simulink model "Simulator_Case_1"  (R2024a)
settings: Solver=VariableStepAuto  StartTime=0.0  StopTime=2842  RelTol=1e-3
values from neighbouring files (symbols this model uses):
  Position_Initial_X = Waypoints_X(1)    [Parametrization_Simulation_Case_1.m]
  Position_Initial_Y = Waypoints_Y(1)    [Parametrization_Simulation_Case_1.m]
undefined symbols (not defined in the file or in its folder): Gain_Derivative_Controller, Gain_Integral_Controller, Gain_Proportional_Controller, Velocity_Ship_Mean, Waypoints
libraries: cstblocks x2
settings Model: Creator=gerar  LastModifiedBy=gerar

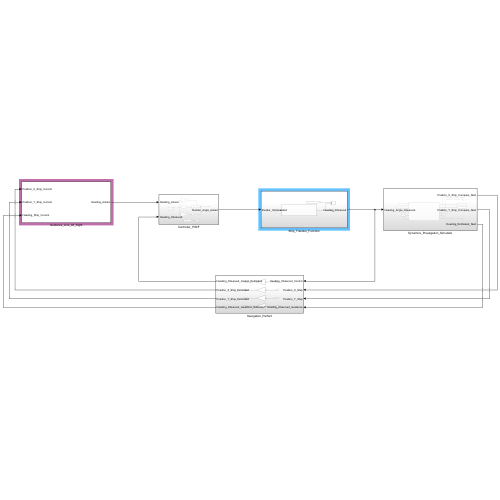
[thumbnail: Simulink's stored preview of the top-level diagram]
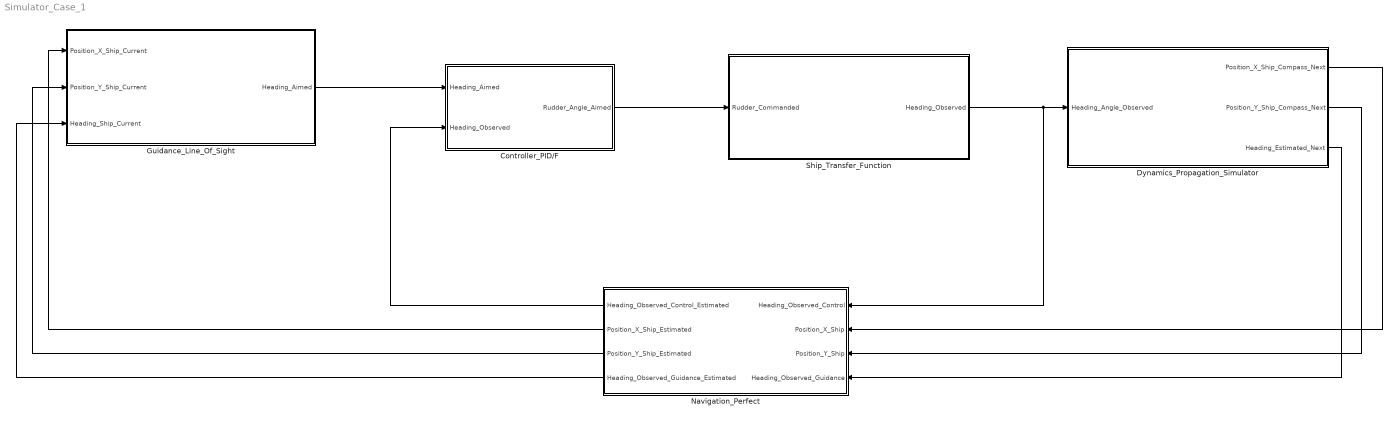
== system Simulator_Case_1 ==
  Controller_PID/F : Subsystem
  Dynamics_Propagation_Simulator : Subsystem
  Guidance_Line_Of_Sight : Subsystem
  Navigation_Perfect : Subsystem
  Ship_Transfer_Function : Subsystem
  wires:
  Guidance_Line_Of_Sight/1(Heading_Aimed) -> Controller_PID/F/1(Heading_Aimed)
  Controller_PID/F/1(Rudder_Angle_Aimed) -> Ship_Transfer_Function/1(Rudder_Commanded)
  Ship_Transfer_Function/1(Heading_Observed) -> Navigation_Perfect/1(Heading_Observed_Control), Dynamics_Propagation_Simulator/1(Heading_Angle_Observed)
  Navigation_Perfect/1(Heading_Observed_Control_Estimated) -> Controller_PID/F/2(Heading_Observed)
  Navigation_Perfect/2(Position_X_Ship_Estimated) -> Guidance_Line_Of_Sight/1(Position_X_Ship_Current)
  Navigation_Perfect/3(Position_Y_Ship_Estimated) -> Guidance_Line_Of_Sight/2(Position_Y_Ship_Current)
  Navigation_Perfect/4(Heading_Observed_Guidance_Estimated) -> Guidance_Line_Of_Sight/3(Heading_Ship_Current)
  Dynamics_Propagation_Simulator/1(Position_X_Ship_Compass_Next) -> Navigation_Perfect/2(Position_X_Ship)
  Dynamics_Propagation_Simulator/2(Position_Y_Ship_Compass_Next) -> Navigation_Perfect/3(Position_Y_Ship)
  Dynamics_Propagation_Simulator/3(Heading_Estimated_Next) -> Navigation_Perfect/4(Heading_Observed_Guidance)

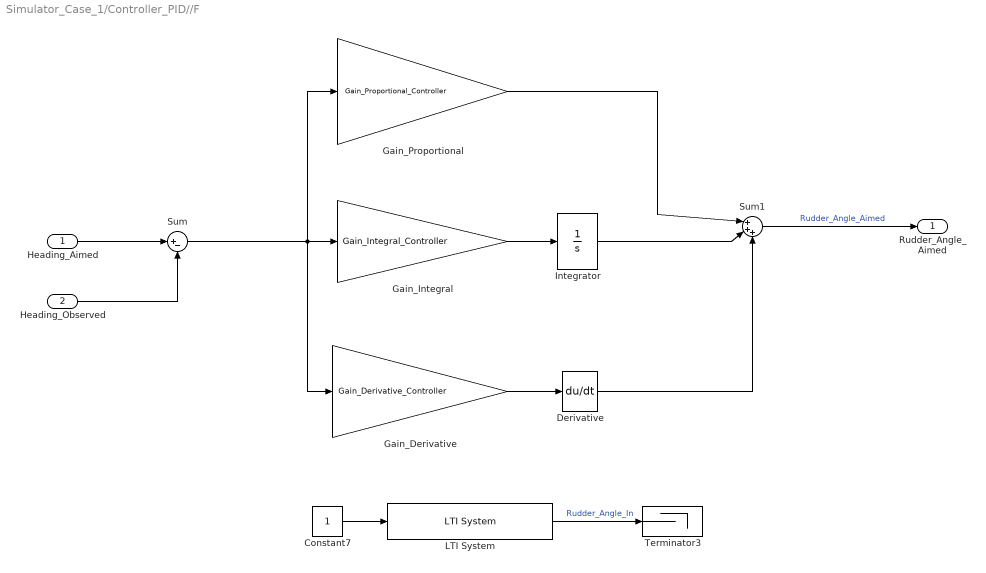
== system Simulator_Case_1/Controller_PID//F ==
  Heading_Aimed : Inport
  Heading_Observed : Inport  Port=2
  Constant7 : Constant
  Derivative : Derivative
  Gain_Derivative : Gain  Gain=Gain_Derivative_Controller
  Gain_Integral : Gain  Gain=Gain_Integral_Controller
  Gain_Proportional : Gain  Gain=Gain_Proportional_Controller
  Integrator : Integrator
  LTI System : cstblocks/LTI System  sys=Controller_PIDF  IC=[]  PadeOrder=0
  Sum : Sum  Inputs=|+-
  Sum1 : Sum  Inputs=|+++
  Terminator3 : Terminator
  Rudder_Angle_Aimed : Outport
  wires:
  Sum/1 -> Gain_Proportional/1, Gain_Integral/1, Gain_Derivative/1
  Gain_Integral/1 -> Integrator/1
  Sum1/1 -> Rudder_Angle_Aimed/1  "Rudder_Angle_Aimed"
  Gain_Proportional/1 -> Sum1/1
  Gain_Derivative/1 -> Derivative/1
  Derivative/1 -> Sum1/3
  Integrator/1 -> Sum1/2
  Heading_Aimed/1 -> Sum/1
  Heading_Observed/1 -> Sum/2
  LTI System/1 -> Terminator3/1  "Rudder_Angle_In"
  Constant7/1 -> LTI System/1

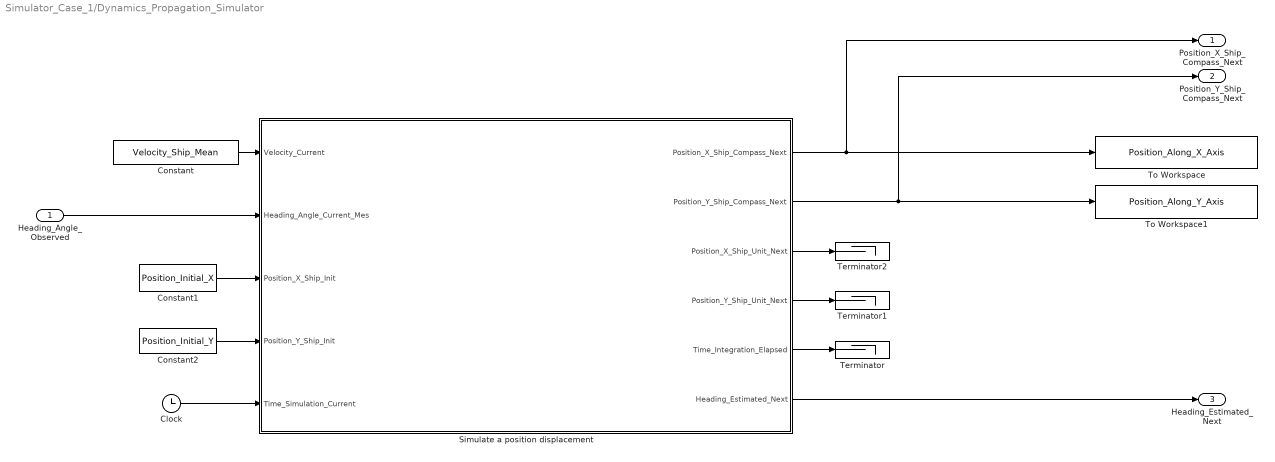
== system Simulator_Case_1/Dynamics_Propagation_Simulator ==
  Heading_Angle_Observed : Inport
  Clock : Clock
  Constant : Constant  Value=Velocity_Ship_Mean
  Constant1 : Constant  Value=Position_Initial_X
  Constant2 : Constant  Value=Position_Initial_Y
  Simulate a position displacement : MATLAB Function  TreatAsAtomicUnit=on
  Terminator : Terminator
  Terminator1 : Terminator
  Terminator2 : Terminator
  To Workspace : ToWorkspace  VariableName=Position_Along_X_Axis  SaveFormat=Timeseries  SampleTime=-1
  To Workspace1 : ToWorkspace  VariableName=Position_Along_Y_Axis  SaveFormat=Timeseries  SampleTime=-1
  Position_X_Ship_Compass_Next : Outport
  Position_Y_Ship_Compass_Next : Outport  Port=2
  Heading_Estimated_Next : Outport  Port=3
  wires:
  Simulate a position displacement/1(Position_X_Ship_Compass_Next) -> Position_X_Ship_Compass_Next/1, To Workspace/1
  Heading_Angle_Observed/1 -> Simulate a position displacement/2(Heading_Angle_Current_Mes)
  Simulate a position displacement/5(Time_Integration_Elapsed) -> Terminator/1
  Simulate a position displacement/4(Position_Y_Ship_Unit_Next) -> Terminator1/1
  Constant1/1 -> Simulate a position displacement/3(Position_X_Ship_Init)
  Constant/1 -> Simulate a position displacement/1(Velocity_Current)
  Simulate a position displacement/2(Position_Y_Ship_Compass_Next) -> Position_Y_Ship_Compass_Next/1, To Workspace1/1
  Simulate a position displacement/3(Position_X_Ship_Unit_Next) -> Terminator2/1
  Constant2/1 -> Simulate a position displacement/4(Position_Y_Ship_Init)
  Clock/1 -> Simulate a position displacement/5(Time_Simulation_Current)
  Simulate a position displacement/6(Heading_Estimated_Next) -> Heading_Estimated_Next/1

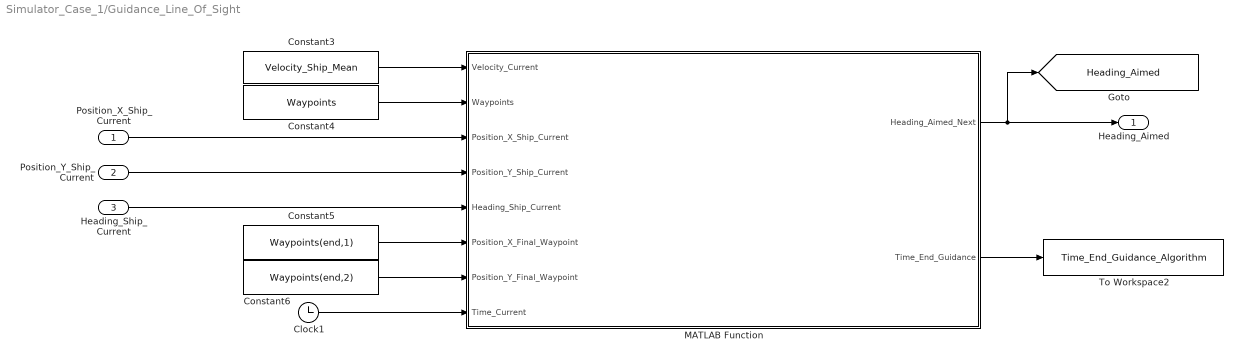
== system Simulator_Case_1/Guidance_Line_Of_Sight ==
  Position_X_Ship_Current : Inport
  Position_Y_Ship_Current : Inport  Port=2
  Heading_Ship_Current : Inport  Port=3
  Clock1 : Clock
  Constant3 : Constant  Value=Velocity_Ship_Mean
  Constant4 : Constant  Value=Waypoints
  Constant5 : Constant  Value=Waypoints(end,1)
  Constant6 : Constant  Value=Waypoints(end,2)
  MATLAB Function : MATLAB Function  TreatAsAtomicUnit=on
  To Workspace2 : ToWorkspace  VariableName=Time_End_Guidance_Algorithm  SaveFormat=Timeseries  SampleTime=-1
  Heading_Aimed : Outport
  tag scope: Heading_Aimed=global
  wires:
  Constant5/1 -> MATLAB Function/6(Position_X_Final_Waypoint)
  Position_X_Ship_Current/1 -> MATLAB Function/3(Position_X_Ship_Current)
  MATLAB Function/1(Heading_Aimed_Next) -> [Heading_Aimed], Heading_Aimed/1
  Constant4/1 -> MATLAB Function/2(Waypoints)
  Constant3/1 -> MATLAB Function/1(Velocity_Current)
  Constant6/1 -> MATLAB Function/7(Position_Y_Final_Waypoint)
  Clock1/1 -> MATLAB Function/8(Time_Current)
  Position_Y_Ship_Current/1 -> MATLAB Function/4(Position_Y_Ship_Current)
  Heading_Ship_Current/1 -> MATLAB Function/5(Heading_Ship_Current)
  MATLAB Function/2(Time_End_Guidance) -> To Workspace2/1

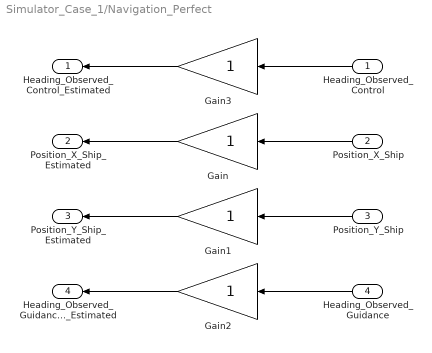
== system Simulator_Case_1/Navigation_Perfect ==
  Heading_Observed_Control : Inport
  Position_X_Ship : Inport  Port=2
  Position_Y_Ship : Inport  Port=3
  Heading_Observed_Guidance : Inport  Port=4
  Gain{,1..3} (4 alike) : Gain
  Heading_Observed_Control_Estimated : Outport
  Position_X_Ship_Estimated : Outport  Port=2
  Position_Y_Ship_Estimated : Outport  Port=3
  Heading_Observed_Guidance_Estimated : Outport  Port=4
  wires:
  Gain1/1 -> Position_Y_Ship_Estimated/1
  Position_X_Ship/1 -> Gain/1
  Heading_Observed_Guidance/1 -> Gain2/1
  Heading_Observed_Control/1 -> Gain3/1
  Gain2/1 -> Heading_Observed_Guidance_Estimated/1
  Position_Y_Ship/1 -> Gain1/1
  Gain/1 -> Position_X_Ship_Estimated/1
  Gain3/1 -> Heading_Observed_Control_Estimated/1

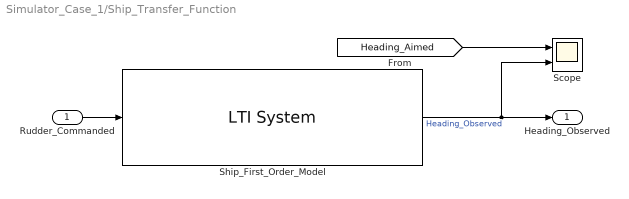
== system Simulator_Case_1/Ship_Transfer_Function ==
  Rudder_Commanded : Inport
  Scope : Scope  NumInputPorts=2
  Ship_First_Order_Model : cstblocks/LTI System  sys=Heading_On_Rudder_Transfer_First_Order  IC=[]  PadeOrder=0
  Heading_Observed : Outport
  wires:
  Ship_First_Order_Model/1 -> Scope/2, Heading_Observed/1  "Heading_Observed"
  Rudder_Commanded/1 -> Ship_First_Order_Model/1
  [Heading_Aimed] -> Scope/1

== matlab function Simulator_Case_1/Guidance_Line_Of_Sight/MATLAB Function ==
  settings: updateMethod=DISCRETE
  data: Velocity_Current input; Heading_Aimed_Next output; Waypoints input; Position_X_Ship_Current input; Position_Y_Ship_Current input; Heading_Ship_Current input; Position_X_Final_Waypoint input; Position_Y_Final_Waypoint input; Time_Current input; Time_End_Guidance output
function [Heading_Aimed_Next,Time_End_Guidance] = Guidance_Waypoints_Following(Velocity_Current,...
                                                                               Waypoints,...
                                                                               Position_X_Ship_Current,...
                                                                               Position_Y_Ship_Current,...
                                                                               Heading_Ship_Current,...
                                                                               Position_X_Final_Waypoint,...
                                                                               Position_Y_Final_Waypoint,...
                                                                               Time_Current)

% Terminal point features:
Position_X_Final_Point = Position_X_Final_Waypoint;
Position_Y_Final_Point = Position_Y_Final_Waypoint;
Radius_Final_Waypoint = 50;

% Enable Guidance to work if the ship is not close to the final waypoint:
if ~((Position_X_Ship_Current - Position_X_Final_Point)^2 + (Position_Y_Ship_Current - Position_Y_Final_Point)^2 <= Radius_Final_Waypoint^2)

    % Then settle the time of end Guidance:
    Time_End_Guidance = 0;

    % Retreive the aimed heading angle that must be performed at this step time
    % of the simulation to follow the Waypoints generated trajectory:
    [Heading_Aimed_Unit,Heading_Aimed_Compass,...
     Heading_Error_Unit,Heading_Error_Compass,...
     Selected_Waypoints,Heading_Current_Unit] = Guidance_Heading_Rudder_Angle(Waypoints,...
                                                                              Position_X_Ship_Current,...
                                                                              Position_Y_Ship_Current, ...
                                                                              Heading_Ship_Current);

else
    
    [Heading_Aimed_Unit,Heading_Aimed_Compass,...
     Heading_Error_Unit,Heading_Error_Compass,...
     Selected_Waypoints,Heading_Current_Unit] = Guidance_Heading_Rudder_Angle(Waypoints,...
                                                                              Position_X_Ship_Current,...
                                                                              Position_Y_Ship_Current, ...
                                                                              Heading_Ship_Current);

    % Then determine the end time of the Guidance scheme:
    Time_End_Guidance = Time_Current;

end

% Then order the heading aimed:
Heading_Aimed_Next = Heading_Aimed_Compass;

end

== matlab function Simulator_Case_1/Dynamics_Propagation_Simulator/Simulate a position displacement ==
  settings: updateMethod=DISCRETE
  data: Velocity_Current input; Position_X_Ship_Compass_Next output; Heading_Angle_Current_Mes input; Position_X_Ship_Init input; Position_Y_Ship_Init input; Time_Simulation_Current input; Position_Y_Ship_Compass_Next output; Position_X_Ship_Unit_Next output; Position_Y_Ship_Unit_Next output; Time_Integration_Elapsed output; Heading_Estimated_Next output
function [Position_X_Ship_Compass_Next,Position_Y_Ship_Compass_Next,...
          Position_X_Ship_Unit_Next,Position_Y_Ship_Unit_Next,...
          Time_Integration_Elapsed,Heading_Estimated_Next] = Position_Propagation(Velocity_Current,Heading_Angle_Current_Mes,...
                                                                                  Position_X_Ship_Init,Position_Y_Ship_Init,...
                                                                                  Time_Simulation_Current)

% Persistents definition:
persistent Position_X_Ship_Compass_Prev
persistent Position_Y_Ship_Compass_Prev
persistent Position_X_Ship_Unit_Prev
persistent Position_Y_Ship_Unit_Prev
persistent Time_Simulation_Previous

% See if the measured heading angle needs conversion to unit circle:
Heading_Angle_Current_Mes_Unit = -Heading_Angle_Current_Mes + (pi/2);

% Simulation time handeling persistent:
if isempty(Time_Simulation_Previous)
    Time_Simulation_Previous = Time_Simulation_Current;
    Time_Integration_Elapsed = Time_Simulation_Current - Time_Simulation_Previous;
else
    Time_Integration_Elapsed = Time_Simulation_Current - Time_Simulation_Previous;
end
Time_Simulation_Previous = Time_Simulation_Current;

% Calculate the local position increment but use both convention (unit and compass):
% Compass:
Position_X_Ship_Current_Increment_Compass = Time_Integration_Elapsed*Velocity_Current*sin(Heading_Angle_Current_Mes);
Position_Y_Ship_Current_Increment_Compass = Time_Integration_Elapsed*Velocity_Current*cos(Heading_Angle_Current_Mes);
% Unit:
Position_X_Ship_Current_Increment_Unit = Time_Integration_Elapsed*Velocity_Current*cos(Heading_Angle_Current_Mes_Unit);
Position_Y_Ship_Current_Increment_Unit = Time_Integration_Elapsed*Velocity_Current*sin(Heading_Angle_Current_Mes_Unit);
% Compass:
if isempty(Position_X_Ship_Compass_Prev)
    Position_X_Ship_Compass_Prev = Position_X_Ship_Init + Position_X_Ship_Current_Increment_Compass;
else
    Position_X_Ship_Compass_Prev = Position_X_Ship_Compass_Prev + Position_X_Ship_Current_Increment_Compass;
end
if isempty(Position_Y_Ship_Compass_Prev)
    Position_Y_Ship_Compass_Prev = Position_Y_Ship_Init + Position_Y_Ship_Current_Increment_Compass;
else
    Position_Y_Ship_Compass_Prev = Position_Y_Ship_Compass_Prev + Position_Y_Ship_Current_Increment_Compass;
end
% Unit:
if isempty(Position_X_Ship_Unit_Prev)
    Position_X_Ship_Unit_Prev = Position_X_Ship_Init + Position_X_Ship_Current_Increment_Unit;
else
    Position_X_Ship_Unit_Prev = Position_X_Ship_Unit_Prev + Position_X_Ship_Current_Increment_Unit;
end
if isempty(Position_Y_Ship_Unit_Prev)
    Position_Y_Ship_Unit_Prev = Position_Y_Ship_Init + Position_Y_Ship_Current_Increment_Unit;
else
    Position_Y_Ship_Unit_Prev = Position_Y_Ship_Unit_Prev + Position_Y_Ship_Current_Increment_Unit;
end

% Then update the persistents:
% Compass:
Position_X_Ship_Compass_Next = Position_X_Ship_Compass_Prev;
Position_Y_Ship_Compass_Next = Position_Y_Ship_Compass_Prev;
% Unit:
Position_X_Ship_Unit_Next = Position_X_Ship_Unit_Prev;
Position_Y_Ship_Unit_Next = Position_Y_Ship_Unit_Prev;

% Just propagate the estimated heading:
Heading_Estimated_Next = Heading_Angle_Current_Mes;

end
